simulink model "Reference_CVS"  (R2026a)
settings: Solver=ode1  StopTime=40
InitFcn:
  | %motor_control_init_m
  | %clear all
  | %close all
  | %clc
  | b=1e-8
  | StepSize = 1e-4;
  | N=1e-17;
  | 
  | VLV_0 =0;%120; %120
  | VA_0 = 0;%300; %300
  | VRV_0 = 0;%130;
  | VP_0 = 0;%500;
  | VLA_0 = 0;%20;
  | VV_0=5000;
  | VRA_0=0;
  | 
  | 
  | QLV_0 = 0;
  | QLA_0 = 0;
  | QP_0 = 0;
  | 
  | bh = 0;
  | th =0;
  | 
  | X_0 = [VLV_0 VA_0 VV_0 VP_0  VLA_0  VRA_0 VRV_0];
  | 
  | 
  | V0 = 10;
  | 
  | K1=.0004;%0.0001
  | K2=0.0009;%0.0009
  | KA=1;%1
  | C1=0.000000003;%0.0000003
  | lambda=6000;%3000
  | X_00 = [VLV_0 VA_0 VV_0 VRV_0];
  | 
  | r2 = 0.05/2;
  | A2 = pi*r2^2;
  | h2 = 0.63;
  | V2 = A2*h2;
  | 
  | 
  | r3 = 0.05/2;
  | A3 = pi*r3^2;
  | h3 = 0.63;
  | V3 = A3*h3;
  | 
  | 
  | rho = 997;
  | gg = 9.81;
  | %
  | init_min=0;
  | init_max=0;
  | %
  | PWM_Period =  StepSize;
  | PWM_Period_g1 = PWM_Period;
  | PWM_Period_g2 =PWM_Period;
  | PWM_Period_g3 = PWM_Period;
  | PWM_Period_g4 = PWM_Period;
  | PWM_Period_g5 = PWM_Period;
  | ... (+158 lines)
libraries: powerlib_meascontrol x12, simulink x8, cstblocks x6
(part 2 of 2)

== system Reference_CVS/Reference CVSs/eRV/eRVhf ==
  note: y = 0,0056x 2 - 0,6667x + 60
  Add18 : Sum
  Add19 : Sum
  Constant20 : Constant  Value=60
  Gain1 : Gain  Gain=1/100
  Gain2 : Gain  Gain=0.0056
  Gain3 : Gain  Gain=-0.6667
  PID : Subsystem  Commented=on
  Product15 : Product
  Scope : Scope
      settings: ActiveDisplayYMinimum=1.07059  ActiveDisplayYMaximum=1.42514
  Stair Generator : powerlib_meascontrol/Pulse & Signal Generators/Stair Generator  Commented=on  t=[0,50,100,150]  e=[3.25,3.5,3.75,4]  Ts=stepsize
      settings: SourceProductName=Simscape Electrical
  Stair Generator1 : powerlib_meascontrol/Pulse & Signal Generators/Stair Generator  Commented=on  t=[100,200,300,400]  e=[3.25,3.5,3.75,4]  Ts=stepsize
      settings: SourceProductName=Simscape Electrical
  Output : Outport
  wires:
  Stair Generator1/1 -> PID/1(s)
  Add19/1 -> Gain1/1
  Gain2/1 -> Add18/1
  Gain3/1 -> Add18/2
  [HR] -> Product15/1, Product15/2, Gain3/1
  Add18/1 -> Add19/1
  Product15/1 -> Gain2/1
  Constant20/1 -> Add19/2
  Gain1/1 -> Scope/1, Output/1

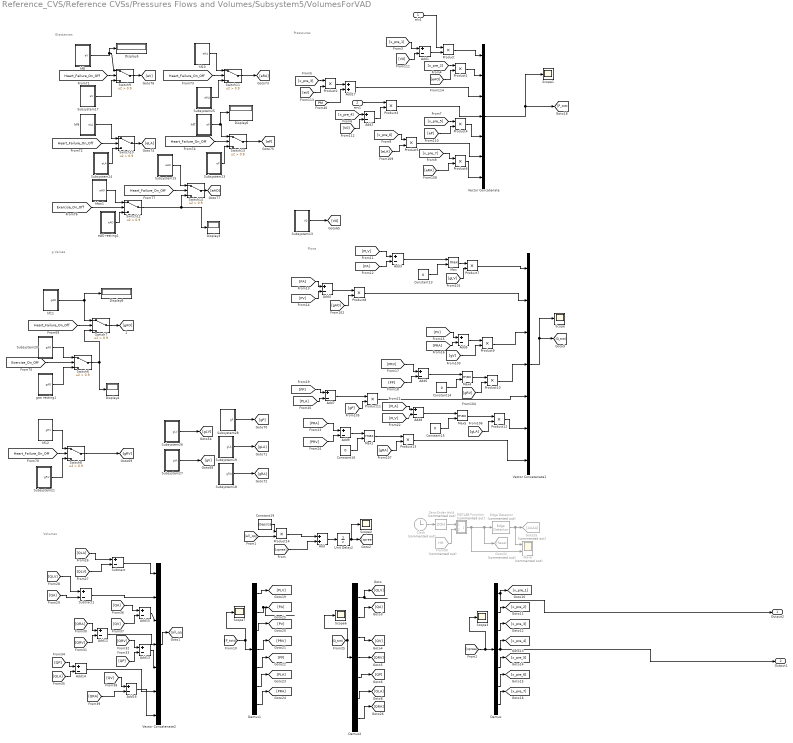
== system Reference_CVS/Reference CVSs/Pressures Flows and Volumes/Subsystem5/VolumesForVAD ==
  note: Elastances
  note: Presssures
  note: g Values
  note: Flows
  note: Volumes
  elv1 : Inport
  erv1 : Inport  Port=2
  Add : Sum
  Add{1..9,12..16} (14 alike) : Sum  Inputs=+-
  Add17 : Sum
  Clock : Clock  Commented=on
      settings: Decimation=10000000
  Constant{13..16} (4 alike) : Constant  Value=0
  Constant19 : Constant  Value=stepsize
  Demux : Demux  Outputs=7
  Demux1 : Demux  Outputs=7
  Demux2 : Demux  Outputs=7
  Display{3..6,8} (5 alike) : Display
  Edge Detector : powerlib_meascontrol/Logic/Edge Detector  Commented=on  model=Falling  ic=0  Ts=0
      settings: SourceProductName=Simscape Electrical
  From90 : From  Commented=on  GotoTag=HR  TagVisibility=global
  Goto32 : Goto  Commented=on  GotoTag=Reset
  Goto55 : Goto  Commented=on  GotoTag=AAAA
  MATLAB Function : MATLAB Function  Commented=on  TreatAsAtomicUnit=on
  Max{,1,4..5} (4 alike) : MinMax  Function=max  Inputs=2
  Product{,1..14} (15 alike) : Product
  Scope{,1..3,6..7} (6 alike) : Scope
      Scope settings: ActiveDisplayYMinimum=-554.9505  ActiveDisplayYMaximum=4972.61734
      Scope1 settings: ActiveDisplayYMinimum=60.37603  ActiveDisplayYMaximum=117.27305  DataLoggingVariableName=ScopeData2
      Scope2 settings: ActiveDisplayYMinimum=-34.04375  ActiveDisplayYMaximum=306.39376  DataLoggingVariableName=ScopeData4
      Scope3 settings: ActiveDisplayYMinimum=-652.22865  ActiveDisplayYMaximum=5628.02541  DataLoggingVariableName=ScopeData5
      Scope6 settings: ActiveDisplayYMinimum=-1063.20433  ActiveDisplayYMaximum=9460.42216  DataLoggingVariableName=ScopeData7
      Scope7 settings: ActiveDisplayYMinimum=-11.3052  ActiveDisplayYMaximum=174.2221  DataLoggingVariableName=ScopeData8
  Subsystem13 : Subsystem
  Subsystem15 : Subsystem
  Subsystem17 : Subsystem
  Subsystem18 : Subsystem
  Subsystem19 : Subsystem
  Subsystem20 : Subsystem
  Subsystem21 : Subsystem
  Subsystem23 : Subsystem
  Subsystem24 : Subsystem
  Subsystem25 : Subsystem
  Subsystem26 : Subsystem
  Subsystem27 : Subsystem
  Subsystem28 : Subsystem
  Subtract : Sum  Inputs=+-
  Subtract1 : Sum  Inputs=+-
  Switch{6..14} (9 alike) : Switch  Criteria=u2 > Threshold  Threshold=0.9  SaturateOnIntegerOverflow=off  InputSameDT=off
  Unit Delay2 : UnitDelay  InitialCondition=X_0  SampleTime=-1
  Vector Concatenate : Concatenate  NumInputs=7
  Vector Concatenate1 : Concatenate  NumInputs=7
  Vector Concatenate2 : Concatenate  NumInputs=7
  Wave : Scope  Commented=on  NumInputPorts=2
      settings: ActiveDisplayYMinimum=-0.125  ActiveDisplayYMaximum=1.125  DataLoggingVariableName=ScopeData10
  Zero-Order Hold : ZeroOrderHold  Commented=on  SampleTime=-1
  eAO resting1 : Subsystem
  gao resting1 : Subsystem
  hf10 : Subsystem
  hf11 : Subsystem
  hf12 : Subsystem
  hf7 : Subsystem
  hf8 : Subsystem
  hf9 : Subsystem
  hfao1 : Subsystem
  Output2 : Outport
  Output1 : Outport  Port=2
  wires:
  Add/1 -> Unit Delay2/1
  Demux1/2 -> [PA]
  Product4/1 -> Vector Concatenate/5
  [QA] -> Add15/1
  Add1/1 -> Product/2
  [P_tott] -> Demux1/1, Scope7/1
  [QRV] -> Add13/1
  Demux/3 -> [x_pre_3]
  [x_pre_7] -> Product6/1
  Product13/1 -> Vector Concatenate1/7
  Demux1/6 -> [PLA]
  [PP] -> Add6/2
  Demux2/2 -> [QA]
  Demux1/4 -> [PRV]
  Product14/1 -> Add/1
  Add9/1 -> Max1/1
  elv1/1 -> Product/1
  Demux2/6 -> [QLA]
  Product/1 -> Vector Concatenate/1
  Constant13/1 -> Max/2
  [QV] -> Add16/1
  [PLV] -> Add8/2
  Constant15/1 -> Max5/2
  [PLV] -> Add3/1
  Max5/1 -> Product12/1
  Demux1/7 -> [PRA]
  [PRV] -> Add6/1
  [PA] -> Add4/1
  Demux1/1 -> [PLV]
  [QRA] -> Add12/1
  [Heart_Failure_On_Off] -> Switch7/2
  [QV] -> Add15/2
  Product10/1 -> Vector Concatenate1/4
  Add5/1 -> Product9/1
  Subsystem21/1(gRV) -> Switch8/3
  Product11/1 -> Vector Concatenate1/5
  [PLA] -> Add8/1
  Add6/1 -> Max4/1
  [PV] -> Add5/1
  [x_pre_4] -> Add2/1
  [QA] -> Subtract1/2
  [x_pre_6] -> Product5/1
  erv1/1 -> Product3/1
  Demux2/1 -> [QLV]
  [x_pre_1] -> Add1/1
  [QRA] -> Add16/2
  [QLA] -> Subtract/1
  Max1/1 -> Product13/1
  Subsystem19/1(gLA) -> [gLA]
  [QLV] -> Subtract1/1
  [Heart_Failure_On_Off] -> Switch10/2
  Add13/1 -> Vector Concatenate2/5
  Add17/1 -> Vector Concatenate/3
  [Heart_Failure_On_Off] -> Switch14/2
  Product9/1 -> Vector Concatenate1/3
  Product2/1 -> Add17/1
  Vector Concatenate/1 -> Scope1/1, [P_tott]
  Unit Delay2/1 -> [xpree], Scope2/1
  Add12/1 -> Vector Concatenate2/4
  hf12/1(gRV) -> Switch8/1
  [x_pre_3] -> Product2/1
  [QLV] -> Subtract/2
  Product3/1 -> Vector Concatenate/4
  [eP] -> Product4/2
  [V0] -> Add2/2
  [gAO] -> Product8/2
  Vector Concatenate1/1 -> Scope/1, [Q_tott]
  Product12/1 -> Vector Concatenate1/6
  [gLA] -> Product12/2
  [gRA] -> Product13/2
  [eV] -> Product2/2
  [eRA] -> Product6/2
  [xpree] -> Add/2
  [gP] -> Product11/2
  Max/1 -> Product7/1
  MATLAB Function/1(y) -> Goto32/1, Edge Detector/1, Wave/2
  Product5/1 -> Vector Concatenate/6
  From90/1 -> MATLAB Function/2(HR)
  [x_pre_5] -> Product4/1
  Switch9/1 -> [eV]
  [gRV] -> Product10/2
  Product8/1 -> Vector Concatenate1/2
  Demux/7 -> [x_pre_7]
  Add8/1 -> Max5/1
  Demux2/7 -> [QRA]
  Vector Concatenate2/1 -> [all_qq]
  Zero-Order Hold/1 -> MATLAB Function/1(u)
  Add15/1 -> Vector Concatenate2/3
  Demux2/5 -> [QP]
  Demux2/4 -> [QRV]
  hfao1/1(eAO) -> Switch12/1
  Add16/1 -> Vector Concatenate2/7
  Max4/1 -> Product10/1
  Edge Detector/1 -> Goto55/1, Wave/1
  Demux/6 -> [x_pre_6]
  Demux/1 -> Output2/1, [x_pre_1]
  [PRA] -> Add9/1
  hf8/1(eV) -> Switch9/1, Display5/1
  Subsystem13/1(V0) -> [V0]
  Subsystem15/1(eAO) -> Switch14/1
  Subsystem27/1(gVt) -> [gV]
  Demux/2 -> [x_pre_2]
  Subsystem26/1(gLV) -> [gLV]
  Add4/1 -> Product8/1
  Add14/1 -> Vector Concatenate2/6
  Demux1/5 -> [PP]
  [PRV] -> Add9/2
  Subtract1/1 -> Vector Concatenate2/2
  [PRA] -> Add5/2
  [QP] -> Add13/2
  [PV] -> Add4/2
  [gV] -> Product9/2
  Switch13/1 -> [eP]
  Clock/1 -> Zero-Order Hold/1
  Switch10/1 -> [eLA]
  [Heart_Failure_On_Off] -> Switch9/2
  [x_pre_2] -> Product1/1
  Add3/1 -> Max/1
  Demux/4 -> Output1/1, [x_pre_4]
  [Heart_Failure_On_Off] -> Switch13/2
  Switch11/1 -> [eRA]
  Switch12/1 -> Switch14/3, Display3/1
  Product7/1 -> Vector Concatenate1/1
  gao resting1/1(gAO) -> Switch6/3
  Switch6/1 -> Display4/1, Switch7/3
  Demux/5 -> [x_pre_5]
  [QP] -> Add14/1
  Constant19/1 -> Product14/1
  Subsystem24/1(eLA) -> Switch10/3
  [PA] -> Add3/2
  ? -> ?
  [PLA] -> Add7/2
  [Heart_Failure_On_Off] -> Switch8/2
  hf11/1(gAO) -> Switch7/1, Display8/1
  Subsystem23/1(eP) -> Switch13/3
  Subsystem17/1(eV) -> Switch9/3
  [eLA] -> Product5/2
  Subsystem20/1(gAO) -> Switch6/1
  Add7/1 -> Product11/1
  [all_qq] -> Product14/2
  Switch14/1 -> [eAO]
  Switch8/1 -> [gRV]
  Subsystem18/1(gRA) -> [gRA]
  Switch7/1 -> [gAO]
  [xpree] -> Demux/1, Scope3/1
  Subsystem28/1(gP) -> [gP]
  Product1/1 -> Vector Concatenate/2
  [PM] -> Add17/2
  hf10/1(eRA) -> Switch11/1
  [QLA] -> Add14/2
  [Exercise_On_Off] -> Switch12/2
  Subtract/1 -> Vector Concatenate2/1
  Demux2/3 -> [QV]
  eAO resting1/1(eAO) -> Switch12/3
  Product6/1 -> Vector Concatenate/7
  [V0] -> Add1/2
  [Heart_Failure_On_Off] -> Switch11/2
  Subsystem25/1(eRA) -> Switch11/3
  [PP] -> Add7/1
  [eAO] -> Product1/2
  Constant14/1 -> Max4/2
  Add2/1 -> Product3/2
  [Q_tott] -> Scope6/1, Demux2/1
  [Exercise_On_Off] -> Switch6/2
  hf9/1(eLA) -> Switch10/1
  Constant16/1 -> Max1/2
  [gLV] -> Product7/2
  [QRV] -> Add12/2
  hf7/1(eP) -> Switch13/1, Display6/1
  Demux1/3 -> [PV]

== system Reference_CVS/Reference CVSs/eLV/LV_e_min/Real_CLV ==
  note: y = 0,2444x 2 - 30,667x + 2560
      | R² = 1
  Add18 : Sum
  Add19 : Sum
  Constant20 : Constant  Value=25600
  Gain : Gain  Gain=1/100
  Gain2 : Gain  Gain=2.444
  Gain3 : Gain  Gain=- 306.67
  Product15 : Product
  C_LV : Outport
  wires:
  Gain/1 -> C_LV/1
  Add18/1 -> Add19/1
  Gain3/1 -> Add18/2
  Product15/1 -> Gain2/1
  Constant20/1 -> Add19/2
  Gain2/1 -> Add18/1
  [HR] -> Product15/1, Product15/2, Gain3/1
  Add19/1 -> Gain/1

== system Reference_CVS/Reference CVSs/eLV/LV_e_min/Subsystem1 ==
  note: y = 0,0446x 2 - 6,3542x + 365,75
      | R² = 1
  Add18 : Sum
  Add19 : Sum
  Constant20 : Constant  Value=365.75
  Gain2 : Gain  Gain=0.0446
  Gain3 : Gain  Gain=- 6.3542
  Product15 : Product
  C_LV : Outport
  wires:
  Add19/1 -> C_LV/1
  [HR] -> Gain3/1, Product15/2, Product15/1
  Gain2/1 -> Add18/1
  Constant20/1 -> Add19/2
  Product15/1 -> Gain2/1
  Gain3/1 -> Add18/2
  Add18/1 -> Add19/1

== system Reference_CVS/Reference CVSs/eLV/LV_e_min/Subsystem2 ==
  note: y = -0,0175x 2 + 5,625x - 264,5
      | R² = 1
  note: y = 0,0011x 2 - 0,4292x + 39,85
      | R² = 1
  note: y = 0,0108x 2 - 4,2917x + 398,5
      | R² = 1
  Add18 : Sum
  Add19 : Sum
  Constant20 : Constant  Value=398.5
  Gain : Gain  Gain=1/10000
  Gain2 : Gain  Gain=0.0108
  Gain3 : Gain  Gain=-4.2917
  Product15 : Product
  Scope : Scope
      settings: ActiveDisplayYMinimum=-0.00112  ActiveDisplayYMaximum=0.02012  DataLoggingVariableName=ScopeData2
  B_LV : Outport
  wires:
  Gain/1 -> B_LV/1, Scope/1
  Add19/1 -> Gain/1
  [HR] -> Gain3/1, Product15/2, Product15/1
  Gain2/1 -> Add18/1
  Constant20/1 -> Add19/2
  Product15/1 -> Gain2/1
  Gain3/1 -> Add18/2
  Add18/1 -> Add19/1

== system Reference_CVS/Reference CVSs/eLV/LV_e_min/Subsystem5 ==
  note: y = -0,0033x 2 + 0,4333x - 2
      | R² = 1
  Add18 : Sum
  Add19 : Sum
  Constant20 : Constant  Value=-20
  Gain : Gain  Gain=1/10000
  Gain2 : Gain  Gain=-0.0333
  Gain3 : Gain  Gain=4.333
  Product15 : Product
  Scope : Scope
      settings: ActiveDisplayYMinimum=-0.00112  ActiveDisplayYMaximum=0.02012  DataLoggingVariableName=ScopeData2
  B_LV_HF : Outport
  wires:
  Add18/1 -> Add19/1
  Gain3/1 -> Add18/2
  Product15/1 -> Gain2/1
  Constant20/1 -> Add19/2
  Gain2/1 -> Add18/1
  [HR] -> Product15/1, Product15/2, Gain3/1
  Add19/1 -> Gain/1
  Gain/1 -> Scope/1, B_LV_HF/1

== system Reference_CVS/Reference CVSs/eLV/LV_e_min/resting ==
  note: y = -4,3333x + 440
  Add19 : Sum
  Constant20 : Constant  Value=440
  Gain : Gain  Gain=1/10000
  Gain3 : Gain  Gain=-4.3333
  Scope : Scope
      settings: ActiveDisplayYMinimum=-0.00112  ActiveDisplayYMaximum=0.02012  DataLoggingVariableName=ScopeData2
  B_LV : Outport
  wires:
  Gain3/1 -> Add19/1
  Constant20/1 -> Add19/2
  [insan] -> Gain3/1
  Add19/1 -> Gain/1
  Gain/1 -> Scope/1, B_LV/1

== system Reference_CVS/Reference CVSs/eLV/eLV1/PID ==
  s : Inport
  LTI System : cstblocks/LTI System  sys=tfa  IC=[]
  PID Controller : simulink/Continuous/PID Controller  Controller=PID  Form=Parallel  TimeDomain=Continuous-time  SampleTime=-1  IntegratorMethod=Forward Euler  FilterMethod=Forward Euler  ControllerParametersSource=internal  P=0  I=0.336541519886425  D=0  UseFilter=on  N=100  TunerSelectOption=Transfer Function Based (PID Tuner App)  InitialConditionSource=internal  InitialConditionForIntegrator=0  InitialConditionForFilter=0  DifferentiatorICPrevScaledInput=0  ExternalReset=none  TrackingMode=off  Kt=1  LimitOutput=off  UpperSaturationLimit=inf  LowerSaturationLimit=-inf  LinearizeAsGain=on  AntiWindupMode=none  Kb=1  POutMin=[]  POutMax=[]  IOutMin=[]  IOutMax=[]  DOutMin=[]  DOutMax=[]  NOutMin=[]  NOutMax=[]  SumOutMin=[]  SumOutMax=[]  SaturationOutMin=[]  SaturationOutMax=[]  PParamMin=[]  PParamMax=[]  IParamMin=[]  IParamMax=[]  DParamMin=[]  DParamMax=[]  NParamMin=[]  NParamMax=[]  KbParamMin=[]  KbParamMax=[]  KtParamMin=[]  KtParamMax=[]  KbOutMin=[]  KbOutMax=[]  KtOutMin=[]  KtOutMax=[]  IntegratorOutMin=[]  IntegratorOutMax=[]  FilterOutMin=[]  FilterOutMax=[]  SumI1OutMin=[]  SumI1OutMax=[]  SumI2OutMin=[]  SumI2OutMax=[]  SumI3OutMin=[]  SumI3OutMax=[]  SumI4OutMin=[]  SumI4OutMax=[]  SumDOutMin=[]  SumDOutMax=[]  DifferentiatorOutMin=[]  DifferentiatorOutMax=[]  FilterDiffOutCoefMin=[]  FilterDiffOutCoefMax=[]  ReciprocalOutMin=[]  ReciprocalOutMax=[]  SumDenOutMin=[]  SumDenOutMax=[]  SumNumOutMin=[]  SumNumOutMax=[]  DivideOutMin=[]  DivideOutMax=[]  IntegratorContinuousStateAttributes=''  IntegratorStateMustResolveToSignalObject=off  IntegratorRTWStateStorageClass=Auto  FilterContinuousStateAttributes=''  FilterStateMustResolveToSignalObject=off  FilterRTWStateStorageClass=Auto  ParallelPVariant=InternalParameters  IdealPVariant=Disabled  IVariant=InternalParameters  DVariant=InternalParameters  IntegratorVariant=Continuous  SatVariant=Disabled  AWVariant=Passthrough  PCopyVariant=Disabled  TRVariant=Disabled  FdbkBlocksVariant=Forward  IdealPFdbkVariant=Disabled  SatFdbkVariant=Disabled  DerivativeFilterVariant=ContFilter  NVariant=InternalParameters  NCopyVariant=Disabled  FilterICVariant=InternalICsFilter  IntegratorICVariant=InternalICs  ExternalResetVariant=Disabled  TRSumVariant=Passthrough  SumFdbkVariant=Disabled  SumVariant=Sum_PID
  Sum1 : Sum  Inputs=|+-
  To Workspace : ToWorkspace  VariableName=input  SampleTime=-1
  To Workspace1 : ToWorkspace  VariableName=output  SampleTime=-1
  E : Outport  VectorParamsAs1DForOutWhenUnconnected=off
  wires:
  PID Controller/1 -> To Workspace/1, LTI System/1
  s/1 -> Sum1/1
  Sum1/1 -> PID Controller/1
  LTI System/1 -> Sum1/2, E/1, To Workspace1/1

== system Reference_CVS/Reference CVSs/eRV/RV_e_min/c_RV ==
  note: y = 0,0167x 2 - 3,3333x + 290
  Add18 : Sum
  Add19 : Sum
  Constant20 : Constant  Value=290
  Gain2 : Gain  Gain=0.0167
  Gain3 : Gain  Gain=-3.3333
  PID : Subsystem  Commented=on
  Product15 : Product
  Scope : Scope
      settings: ActiveDisplayYMinimum=1.07059  ActiveDisplayYMaximum=1.42514
  Stair Generator : powerlib_meascontrol/Pulse & Signal Generators/Stair Generator  Commented=on  t=[0,50,100,150]  e=[3.25,3.5,3.75,4]  Ts=stepsize
      settings: SourceProductName=Simscape Electrical
  Stair Generator1 : powerlib_meascontrol/Pulse & Signal Generators/Stair Generator  Commented=on  t=[100,200,300,400]  e=[3.25,3.5,3.75,4]  Ts=stepsize
      settings: SourceProductName=Simscape Electrical
  Output : Outport
  wires:
  Add19/1 -> Output/1, Scope/1
  Constant20/1 -> Add19/2
  Product15/1 -> Gain2/1
  Add18/1 -> Add19/1
  [HR] -> Gain3/1, Product15/2, Product15/1
  Gain3/1 -> Add18/2
  Gain2/1 -> Add18/1
  Stair Generator1/1 -> PID/1(s)

== system Reference_CVS/Reference CVSs/eRV/RV_e_min/real_c_RV ==
  note: y = - 333,33x + 110000
      | R² = 1
  Add19 : Sum
  Constant20 : Constant  Value=110000
  Gain1 : Gain  Gain=1/1000
  Gain3 : Gain  Gain=-333.33
  PID : Subsystem  Commented=on
  Scope : Scope
      settings: ActiveDisplayYMinimum=1.07059  ActiveDisplayYMaximum=1.42514
  Stair Generator : powerlib_meascontrol/Pulse & Signal Generators/Stair Generator  Commented=on  t=[0,50,100,150]  e=[3.25,3.5,3.75,4]  Ts=stepsize
      settings: SourceProductName=Simscape Electrical
  Stair Generator1 : powerlib_meascontrol/Pulse & Signal Generators/Stair Generator  Commented=on  t=[100,200,300,400]  e=[3.25,3.5,3.75,4]  Ts=stepsize
      settings: SourceProductName=Simscape Electrical
  Output : Outport
  wires:
  Gain1/1 -> Scope/1, Output/1
  Stair Generator1/1 -> PID/1(s)
  [HR] -> Gain3/1
  Gain3/1 -> Add19/1
  Constant20/1 -> Add19/2
  Add19/1 -> Gain1/1

== system Reference_CVS/Reference CVSs/eRV/Subsystem2/k_0 ==
  note: y = -0,0042x 2 - 0,0417x + 257,5
      | R² = 1
  In1 : Inport
  Add4 : Sum
  Add5 : Sum
  Constant4 : Constant  Value=257.5
  Gain : Gain  Gain=-0.0041
  Gain1 : Gain  Gain=-0.0417
  Multiply : Gain  Gain=1/1000
  Product8 : Product
  Out1 : Outport
  wires:
  Multiply/1 -> Out1/1
  Add5/1 -> Multiply/1
  Constant4/1 -> Add5/2
  Gain/1 -> Add4/1
  Gain1/1 -> Add4/2
  Product8/1 -> Gain/1
  In1/1 -> Product8/1, Product8/2, Gain1/1
  Add4/1 -> Add5/1

== system Reference_CVS/Reference CVSs/eRV/Subsystem2/k_1 ==
  note: y = 0,0158x 2 - 5,0417x + 445,5
      | R² = 1
  In1 : Inport
  Add6 : Sum
  Add7 : Sum
  Constant7 : Constant  Value=445.5
  Gain2 : Gain  Gain=0.0158
  Gain3 : Gain  Gain=-5.0417
  Multiply : Gain  Gain=1/1000
  Product10 : Product
  Out1 : Outport
  wires:
  Multiply/1 -> Out1/1
  Add7/1 -> Multiply/1
  Product10/1 -> Gain2/1
  Add6/1 -> Add7/1
  Gain3/1 -> Add6/2
  In1/1 -> Product10/1, Product10/2, Gain3/1
  Gain2/1 -> Add6/1
  Constant7/1 -> Add7/2

== system Reference_CVS/Reference CVSs/eRV/eRV2/PID ==
  s : Inport
  LTI System : cstblocks/LTI System  sys=tfa  IC=[]
  PID Controller : simulink/Continuous/PID Controller  Controller=PID  Form=Parallel  TimeDomain=Continuous-time  SampleTime=-1  IntegratorMethod=Forward Euler  FilterMethod=Forward Euler  ControllerParametersSource=internal  P=0  I=0.336541519886425  D=0  UseFilter=on  N=100  TunerSelectOption=Transfer Function Based (PID Tuner App)  InitialConditionSource=internal  InitialConditionForIntegrator=0  InitialConditionForFilter=0  DifferentiatorICPrevScaledInput=0  ExternalReset=none  TrackingMode=off  Kt=1  LimitOutput=off  UpperSaturationLimit=inf  LowerSaturationLimit=-inf  LinearizeAsGain=on  AntiWindupMode=none  Kb=1  POutMin=[]  POutMax=[]  IOutMin=[]  IOutMax=[]  DOutMin=[]  DOutMax=[]  NOutMin=[]  NOutMax=[]  SumOutMin=[]  SumOutMax=[]  SaturationOutMin=[]  SaturationOutMax=[]  PParamMin=[]  PParamMax=[]  IParamMin=[]  IParamMax=[]  DParamMin=[]  DParamMax=[]  NParamMin=[]  NParamMax=[]  KbParamMin=[]  KbParamMax=[]  KtParamMin=[]  KtParamMax=[]  KbOutMin=[]  KbOutMax=[]  KtOutMin=[]  KtOutMax=[]  IntegratorOutMin=[]  IntegratorOutMax=[]  FilterOutMin=[]  FilterOutMax=[]  SumI1OutMin=[]  SumI1OutMax=[]  SumI2OutMin=[]  SumI2OutMax=[]  SumI3OutMin=[]  SumI3OutMax=[]  SumI4OutMin=[]  SumI4OutMax=[]  SumDOutMin=[]  SumDOutMax=[]  DifferentiatorOutMin=[]  DifferentiatorOutMax=[]  FilterDiffOutCoefMin=[]  FilterDiffOutCoefMax=[]  ReciprocalOutMin=[]  ReciprocalOutMax=[]  SumDenOutMin=[]  SumDenOutMax=[]  SumNumOutMin=[]  SumNumOutMax=[]  DivideOutMin=[]  DivideOutMax=[]  IntegratorContinuousStateAttributes=''  IntegratorStateMustResolveToSignalObject=off  IntegratorRTWStateStorageClass=Auto  FilterContinuousStateAttributes=''  FilterStateMustResolveToSignalObject=off  FilterRTWStateStorageClass=Auto  ParallelPVariant=InternalParameters  IdealPVariant=Disabled  IVariant=InternalParameters  DVariant=InternalParameters  IntegratorVariant=Continuous  SatVariant=Disabled  AWVariant=Passthrough  PCopyVariant=Disabled  TRVariant=Disabled  FdbkBlocksVariant=Forward  IdealPFdbkVariant=Disabled  SatFdbkVariant=Disabled  DerivativeFilterVariant=ContFilter  NVariant=InternalParameters  NCopyVariant=Disabled  FilterICVariant=InternalICsFilter  IntegratorICVariant=InternalICs  ExternalResetVariant=Disabled  TRSumVariant=Passthrough  SumFdbkVariant=Disabled  SumVariant=Sum_PID
  Sum1 : Sum  Inputs=|+-
  To Workspace : ToWorkspace  VariableName=input  SampleTime=-1
  To Workspace1 : ToWorkspace  VariableName=output  SampleTime=-1
  E : Outport  VectorParamsAs1DForOutWhenUnconnected=off
  wires:
  LTI System/1 -> To Workspace1/1, E/1, Sum1/2
  Sum1/1 -> PID Controller/1
  s/1 -> Sum1/1
  PID Controller/1 -> LTI System/1, To Workspace/1

== system Reference_CVS/Reference CVSs/eRV/eRVhf/PID ==
  s : Inport
  LTI System : cstblocks/LTI System  sys=tfa  IC=[]
  PID Controller : simulink/Continuous/PID Controller  Controller=PID  Form=Parallel  TimeDomain=Continuous-time  SampleTime=-1  IntegratorMethod=Forward Euler  FilterMethod=Forward Euler  ControllerParametersSource=internal  P=0  I=0.336541519886425  D=0  UseFilter=on  N=100  TunerSelectOption=Transfer Function Based (PID Tuner App)  InitialConditionSource=internal  InitialConditionForIntegrator=0  InitialConditionForFilter=0  DifferentiatorICPrevScaledInput=0  ExternalReset=none  TrackingMode=off  Kt=1  LimitOutput=off  UpperSaturationLimit=inf  LowerSaturationLimit=-inf  LinearizeAsGain=on  AntiWindupMode=none  Kb=1  POutMin=[]  POutMax=[]  IOutMin=[]  IOutMax=[]  DOutMin=[]  DOutMax=[]  NOutMin=[]  NOutMax=[]  SumOutMin=[]  SumOutMax=[]  SaturationOutMin=[]  SaturationOutMax=[]  PParamMin=[]  PParamMax=[]  IParamMin=[]  IParamMax=[]  DParamMin=[]  DParamMax=[]  NParamMin=[]  NParamMax=[]  KbParamMin=[]  KbParamMax=[]  KtParamMin=[]  KtParamMax=[]  KbOutMin=[]  KbOutMax=[]  KtOutMin=[]  KtOutMax=[]  IntegratorOutMin=[]  IntegratorOutMax=[]  FilterOutMin=[]  FilterOutMax=[]  SumI1OutMin=[]  SumI1OutMax=[]  SumI2OutMin=[]  SumI2OutMax=[]  SumI3OutMin=[]  SumI3OutMax=[]  SumI4OutMin=[]  SumI4OutMax=[]  SumDOutMin=[]  SumDOutMax=[]  DifferentiatorOutMin=[]  DifferentiatorOutMax=[]  FilterDiffOutCoefMin=[]  FilterDiffOutCoefMax=[]  ReciprocalOutMin=[]  ReciprocalOutMax=[]  SumDenOutMin=[]  SumDenOutMax=[]  SumNumOutMin=[]  SumNumOutMax=[]  DivideOutMin=[]  DivideOutMax=[]  IntegratorContinuousStateAttributes=''  IntegratorStateMustResolveToSignalObject=off  IntegratorRTWStateStorageClass=Auto  FilterContinuousStateAttributes=''  FilterStateMustResolveToSignalObject=off  FilterRTWStateStorageClass=Auto  ParallelPVariant=InternalParameters  IdealPVariant=Disabled  IVariant=InternalParameters  DVariant=InternalParameters  IntegratorVariant=Continuous  SatVariant=Disabled  AWVariant=Passthrough  PCopyVariant=Disabled  TRVariant=Disabled  FdbkBlocksVariant=Forward  IdealPFdbkVariant=Disabled  SatFdbkVariant=Disabled  DerivativeFilterVariant=ContFilter  NVariant=InternalParameters  NCopyVariant=Disabled  FilterICVariant=InternalICsFilter  IntegratorICVariant=InternalICs  ExternalResetVariant=Disabled  TRSumVariant=Passthrough  SumFdbkVariant=Disabled  SumVariant=Sum_PID
  Sum1 : Sum  Inputs=|+-
  To Workspace : ToWorkspace  VariableName=input  SampleTime=-1
  To Workspace1 : ToWorkspace  VariableName=output  SampleTime=-1
  E : Outport  VectorParamsAs1DForOutWhenUnconnected=off
  wires:
  LTI System/1 -> To Workspace1/1, E/1, Sum1/2
  Sum1/1 -> PID Controller/1
  s/1 -> Sum1/1
  PID Controller/1 -> LTI System/1, To Workspace/1

== system Reference_CVS/Reference CVSs/Pressures Flows and Volumes/Subsystem5/VolumesForVAD/Subsystem13 ==
  note: y = 0,1944x 2 - 28,333x + 1100
  Add{1..2,18..19} (4 alike) : Sum
  Constant1 : Constant  Value=2750
  Constant20 : Constant  Value=1100
  Display : Display
  Gain : Gain  Gain=1/10
  Gain1 : Gain  Gain=1/1000
  Gain2 : Gain  Gain=0.1944
  Gain3 : Gain  Gain=-28.333
  Gain4 : Gain  Gain=-0.4167
  Gain5 : Gain  Gain=145.83
  Product1 : Product
  Product15 : Product
  Scope : Scope
      settings: ActiveDisplayYMinimum=8.99968  ActiveDisplayYMaximum=10.99968  DataLoggingVariableName=ScopeData2
  Scope1 : Scope
      settings: ActiveDisplayYMinimum=8.99968  ActiveDisplayYMaximum=10.99968
  Switch : Switch  Criteria=u2 > Threshold  SaturateOnIntegerOverflow=off  InputSameDT=off
  V0 : Outport
  wires:
  Switch/1 -> V0/1, Display/1
  [Heart_Failure_On_Off] -> Switch/2
  Add2/1 -> Gain1/1
  Add1/1 -> Add2/1
  Gain5/1 -> Add1/2
  Product1/1 -> Gain4/1
  Constant1/1 -> Add2/2
  Gain4/1 -> Add1/1
  [HR] -> Product1/1, Product1/2, Gain5/1
  Gain1/1 -> Scope1/1, Switch/3
  Gain/1 -> Scope/1, Switch/1
  [HR] -> Gain3/1, Product15/2, Product15/1
  Gain2/1 -> Add18/1
  Constant20/1 -> Add19/2
  Product15/1 -> Gain2/1
  Gain3/1 -> Add18/2
  Add18/1 -> Add19/1
  Add19/1 -> Gain/1

== system Reference_CVS/Reference CVSs/Pressures Flows and Volumes/Subsystem5/VolumesForVAD/Subsystem15 ==
  note: y = -0,0278x 2 + 5,8333x - 150
  Add18 : Sum
  Add19 : Sum
  Constant20 : Constant  Value=-150
  Gain2 : Gain  Gain=-0.0278
  Gain3 : Gain  Gain=5.8333
  Multiply : Gain  Gain=1/100
  Product15 : Product
  Scope : Scope
      settings: ActiveDisplayYMinimum=0.50527  ActiveDisplayYMaximum=0.53249  DataLoggingVariableName=ScopeData2
  eAO : Outport
  wires:
  Multiply/1 -> Scope/1, eAO/1
  [HR] -> Gain3/1, Product15/2, Product15/1
  Gain2/1 -> Add18/1
  Constant20/1 -> Add19/2
  Product15/1 -> Gain2/1
  Gain3/1 -> Add18/2
  Add18/1 -> Add19/1
  Add19/1 -> Multiply/1

== system Reference_CVS/Reference CVSs/Pressures Flows and Volumes/Subsystem5/VolumesForVAD/Subsystem17 ==
  note: y = -0,0033x 2 + 0,8667x - 16
  Add18 : Sum
  Add19 : Sum
  Constant20 : Constant  Value=-16
  Gain1 : Gain  Gain=1/10000
  Gain2 : Gain  Gain=-0.0033
  Gain3 : Gain  Gain=0.8667
  Product15 : Product
  Scope : Scope
      settings: ActiveDisplayYMinimum=0.00132  ActiveDisplayYMaximum=0.00154  DataLoggingVariableName=ScopeData2
  eV : Outport
  wires:
  Add18/1 -> Add19/1
  Gain3/1 -> Add18/2
  Product15/1 -> Gain2/1
  Constant20/1 -> Add19/2
  Gain2/1 -> Add18/1
  [HR] -> Product15/1, Product15/2, Gain3/1
  Add19/1 -> Gain1/1
  Gain1/1 -> Scope/1, eV/1

== system Reference_CVS/Reference CVSs/Pressures Flows and Volumes/Subsystem5/VolumesForVAD/Subsystem18 ==
  note: y = 0,0167x 2 - 5,8333x + 1290
      | R² = 1
  Add19 : Sum
  Constant20 : Constant  Value=1150
  Gain3 : Gain  Gain=-2.5
  Scope : Scope
      settings: ActiveDisplayYMinimum=900  ActiveDisplayYMaximum=1100  DataLoggingVariableName=ScopeData2
  gRA : Outport
  wires:
  Gain3/1 -> Add19/1
  Add19/1 -> gRA/1, Scope/1
  [HR] -> Gain3/1
  Constant20/1 -> Add19/2

== system Reference_CVS/Reference CVSs/Pressures Flows and Volumes/Subsystem5/VolumesForVAD/Subsystem19 ==
  note: y = 0,0167x 2 - 5,8333x + 1290
      | R² = 1
  note: y = - 5x + 1300R² = 1
  Add19 : Sum
  Constant20 : Constant  Value=1300
  Gain3 : Gain  Gain=-5
  Scope : Scope
      settings: ActiveDisplayYMinimum=900  ActiveDisplayYMaximum=1100  DataLoggingVariableName=ScopeData2
  gLA : Outport
  wires:
  Gain3/1 -> Add19/1
  Constant20/1 -> Add19/2
  [HR] -> Gain3/1
  Add19/1 -> Scope/1, gLA/1

== system Reference_CVS/Reference CVSs/Pressures Flows and Volumes/Subsystem5/VolumesForVAD/Subsystem20 ==
  note: y = 0,0058x 2 + 1,4583x - 18,5
  Add18 : Sum
  Add19 : Sum
  Constant20 : Constant  Value=-18.5
  Gain1 : Gain  Gain=1/100
  Gain2 : Gain  Gain=0.0058
  Gain3 : Gain  Gain=1.4583
  Product15 : Product
  Scope : Scope
      settings: ActiveDisplayYMinimum=0.88246  ActiveDisplayYMaximum=1.08246  DataLoggingVariableName=ScopeData2
  gAO : Outport
  wires:
  Add18/1 -> Add19/1
  Gain3/1 -> Add18/2
  Product15/1 -> Gain2/1
  Constant20/1 -> Add19/2
  Gain2/1 -> Add18/1
  [HR] -> Product15/1, Product15/2, Gain3/1
  Add19/1 -> Gain1/1
  Gain1/1 -> Scope/1, gAO/1

== system Reference_CVS/Reference CVSs/Pressures Flows and Volumes/Subsystem5/VolumesForVAD/Subsystem21 ==
  note: y = 0,0742x 2 - 10,958x + 600,5
  Add18 : Sum
  Add19 : Sum
  Constant20 : Constant  Value=600.5
  Gain : Gain
  Gain2 : Gain  Gain=0.0742
  Gain3 : Gain  Gain=-10.958
  Product15 : Product
  Scope : Scope
      settings: ActiveDisplayYMinimum=109.99968  ActiveDisplayYMaximum=309.99968  DataLoggingVariableName=ScopeData2
  gRV : Outport
  wires:
  Add19/1 -> Gain/1
  [HR] -> Gain3/1, Product15/2, Product15/1
  Gain2/1 -> Add18/1
  Constant20/1 -> Add19/2
  Product15/1 -> Gain2/1
  Gain3/1 -> Add18/2
  Add18/1 -> Add19/1
  Gain/1 -> gRV/1, Scope/1

== system Reference_CVS/Reference CVSs/Pressures Flows and Volumes/Subsystem5/VolumesForVAD/Subsystem23 ==
  note: y = 0,1417x 2 - 24,583x + 2165
  Add18 : Sum
  Add19 : Sum
  Constant20 : Constant  Value=2165
  Gain : Gain  Gain=1/10000
  Gain2 : Gain  Gain=0.1417
  Gain3 : Gain  Gain=-24.583
  Product15 : Product
  Scope : Scope
      settings: ActiveDisplayYMinimum=0.01994  ActiveDisplayYMaximum=0.21994  DataLoggingVariableName=ScopeData2
  eP : Outport
  wires:
  Add19/1 -> Gain/1
  [HR] -> Gain3/1, Product15/2, Product15/1
  Gain2/1 -> Add18/1
  Constant20/1 -> Add19/2
  Product15/1 -> Gain2/1
  Gain3/1 -> Add18/2
  Add18/1 -> Add19/1
  Gain/1 -> eP/1, Scope/1

== system Reference_CVS/Reference CVSs/Pressures Flows and Volumes/Subsystem5/VolumesForVAD/Subsystem24 ==
  note: y = -0,0069x2 + 1,2813x + 30,375R² = 1
  note: y = -2E-06x 2 + 0,0011x + 0,044
      | R² = 1
  Add18 : Sum
  Add19 : Sum
  Constant20 : Constant  Value=30.375
  Gain : Gain  Gain=1/1000
  Gain2 : Gain  Gain=-0.0069
  Gain3 : Gain  Gain=1.2813
  Product15 : Product
  Scope : Scope
      settings: ActiveDisplayYMinimum=0.07241  ActiveDisplayYMaximum=0.09241  DataLoggingVariableName=ScopeData2
  eLA : Outport
  wires:
  Add18/1 -> Add19/1
  Gain3/1 -> Add18/2
  Product15/1 -> Gain2/1
  Constant20/1 -> Add19/2
  Gain2/1 -> Add18/1
  [HR] -> Product15/1, Product15/2, Gain3/1
  Add19/1 -> Gain/1
  Gain/1 -> eLA/1, Scope/1

== system Reference_CVS/Reference CVSs/Pressures Flows and Volumes/Subsystem5/VolumesForVAD/Subsystem25 ==
  note: y = -0,1479x 2 + 38,021x - 923,75
  Add18 : Sum
  Add19 : Sum
  Constant20 : Constant  Value=-923.75
  Gain : Gain  Gain=1/10000
  Gain2 : Gain  Gain=-0.1479
  Gain3 : Gain  Gain=38.021
  Product15 : Product
  Scope : Scope
      settings: ActiveDisplayYMinimum=0.07241  ActiveDisplayYMaximum=0.09241
  eRA : Outport
  wires:
  Gain/1 -> eRA/1, Scope/1
  Gain2/1 -> Add18/1
  Gain3/1 -> Add18/2
  Product15/1 -> Gain2/1
  Add18/1 -> Add19/1
  Constant20/1 -> Add19/2
  [HR] -> Product15/1, Product15/2, Gain3/1
  Add19/1 -> Gain/1

== system Reference_CVS/Reference CVSs/Pressures Flows and Volumes/Subsystem5/VolumesForVAD/Subsystem26 ==
  note: y = 4,1667x2 + 3041,7x + 12500R² = 1
  note: y = -0,0225x 2 + 8,375x - 211,5
      | R² = 1
  Add18 : Sum
  Add19 : Sum
  Constant20 : Constant  Value=12500
  Gain : Gain  Gain=1/1000
  Gain2 : Gain  Gain=4.1667
  Gain3 : Gain  Gain=3041.7
  Product15 : Product
  Scope : Scope
      settings: ActiveDisplayYMinimum=197.50212  ActiveDisplayYMaximum=216.59303  DataLoggingVariableName=ScopeData2
  gLV : Outport
  wires:
  Add19/1 -> Gain/1
  [HR] -> Gain3/1, Product15/2, Product15/1
  Gain2/1 -> Add18/1
  Constant20/1 -> Add19/2
  Product15/1 -> Gain2/1
  Gain3/1 -> Add18/2
  Add18/1 -> Add19/1
  Gain/1 -> gLV/1, Scope/1

== system Reference_CVS/Reference CVSs/Pressures Flows and Volumes/Subsystem5/VolumesForVAD/Subsystem27 ==
  note: y = 0,25x2 + 1212,5x - 3650R² = 1
  note: y = -0,0092x 2 + 3,2083x - 89,5
      | R² = 1
  Add18 : Sum
  Add19 : Sum
  Constant20 : Constant  Value=-3650
  Gain : Gain  Gain=1/1000
  Gain2 : Gain  Gain=0.25
  Gain3 : Gain  Gain=1212.5
  Product15 : Product
  Scope : Scope
      settings: ActiveDisplayYMinimum=60  ActiveDisplayYMaximum=80  DataLoggingVariableName=ScopeData2
  gVt : Outport
  wires:
  Add19/1 -> Gain/1
  [HR] -> Gain3/1, Product15/2, Product15/1
  Gain2/1 -> Add18/1
  Constant20/1 -> Add19/2
  Product15/1 -> Gain2/1
  Gain3/1 -> Add18/2
  Add18/1 -> Add19/1
  Gain/1 -> gVt/1, Scope/1

== system Reference_CVS/Reference CVSs/Pressures Flows and Volumes/Subsystem5/VolumesForVAD/Subsystem28 ==
  note: y = -0,0208x 2 + 4,7917x - 162,5
  Add18 : Sum
  Add19 : Sum
  Constant20 : Constant  Value=-162.5
  Gain : Gain  Gain=1/10
  Gain2 : Gain  Gain=-0.0208
  Gain3 : Gain  Gain=4.7917
  Product15 : Product
  Scope : Scope
      settings: ActiveDisplayYMinimum=3.9997  ActiveDisplayYMaximum=5.9997  DataLoggingVariableName=ScopeData2
  gP : Outport
  wires:
  Add18/1 -> Add19/1
  Gain3/1 -> Add18/2
  Product15/1 -> Gain2/1
  Constant20/1 -> Add19/2
  Gain2/1 -> Add18/1
  [HR] -> Product15/1, Product15/2, Gain3/1
  Add19/1 -> Gain/1
  Gain/1 -> Scope/1, gP/1

== system Reference_CVS/Reference CVSs/Pressures Flows and Volumes/Subsystem5/VolumesForVAD/eAO resting1 ==
  note: y = 0,5x + 40
  Add19 : Sum
  Constant20 : Constant  Value=40
  Gain1 : Gain  Gain=1/100
  Gain3 : Gain  Gain=0.5
  Scope : Scope
      settings: ActiveDisplayYMinimum=0.50527  ActiveDisplayYMaximum=0.53249  DataLoggingVariableName=ScopeData2
  eAO : Outport
  wires:
  Add19/1 -> Gain1/1
  Gain3/1 -> Add19/1
  Constant20/1 -> Add19/2
  [insan] -> Gain3/1
  Gain1/1 -> eAO/1, Scope/1

== system Reference_CVS/Reference CVSs/Pressures Flows and Volumes/Subsystem5/VolumesForVAD/gao resting1 ==
  note: y = -0,0167x 2 + 3,25x - 45
  Add18 : Sum
  Add19 : Sum
  Constant20 : Constant  Value=-45
  Gain1 : Gain  Gain=1/100
  Gain2 : Gain  Gain=-0.0167
  Gain3 : Gain  Gain=3.25
  Product15 : Product
  Scope : Scope
      settings: ActiveDisplayYMinimum=0.88246  ActiveDisplayYMaximum=1.08246  DataLoggingVariableName=ScopeData2
  gAO : Outport
  wires:
  Gain1/1 -> gAO/1, Scope/1
  Add19/1 -> Gain1/1
  [insan] -> Gain3/1, Product15/2, Product15/1
  Gain2/1 -> Add18/1
  Constant20/1 -> Add19/2
  Product15/1 -> Gain2/1
  Gain3/1 -> Add18/2
  Add18/1 -> Add19/1

== system Reference_CVS/Reference CVSs/Pressures Flows and Volumes/Subsystem5/VolumesForVAD/hf10 ==
  note: y = -0,0069x2 + 1,2813x + 30,375R² = 1
  note: y = -2E-06x 2 + 0,0011x + 0,044
      | R² = 1
  note: y = 0,015x 2 - 2,25x + 301
  Add18 : Sum
  Add19 : Sum
  Constant20 : Constant  Value=301
  Gain : Gain  Gain=1/1000
  Gain2 : Gain  Gain=0.015
  Gain3 : Gain  Gain=-2.25
  Product15 : Product
  Scope : Scope
      settings: ActiveDisplayYMinimum=0.07241  ActiveDisplayYMaximum=0.09241
  eRA : Outport
  wires:
  Add19/1 -> Gain/1
  [HR] -> Gain3/1, Product15/2, Product15/1
  Constant20/1 -> Add19/2
  Add18/1 -> Add19/1
  Product15/1 -> Gain2/1
  Gain3/1 -> Add18/2
  Gain2/1 -> Add18/1
  Gain/1 -> Scope/1, eRA/1

== system Reference_CVS/Reference CVSs/Pressures Flows and Volumes/Subsystem5/VolumesForVAD/hf11 ==
  note: y = -0,0014x 2 + 0,4834x - 14,119
      | R² = 1
  note: y = -0,0073x2 + 26,677x - 591,88R² = 1
  note: y = 0,0079x 2 - 0,7958x + 117,5
  Add18 : Sum
  Add19 : Sum
  Constant20 : Constant  Value=117.5
  Gain1 : Gain  Gain=1/100
  Gain2 : Gain  Gain=0.0079
  Gain3 : Gain  Gain=-0.7958
  Product15 : Product
  Scope : Scope
      settings: ActiveDisplayYMinimum=0.88246  ActiveDisplayYMaximum=1.08246  DataLoggingVariableName=ScopeData2
  gAO : Outport
  wires:
  Gain1/1 -> gAO/1, Scope/1
  Add19/1 -> Gain1/1
  [HR] -> Gain3/1, Product15/2, Product15/1
  Gain2/1 -> Add18/1
  Constant20/1 -> Add19/2
  Product15/1 -> Gain2/1
  Gain3/1 -> Add18/2
  Add18/1 -> Add19/1

== system Reference_CVS/Reference CVSs/Pressures Flows and Volumes/Subsystem5/VolumesForVAD/hf12 ==
  note: y = -0,0008x 2 + 0,2917x + 195,5
      | R² = 1
  note: y = -0,1667x2 + 158,33x + 201100R² = 1
  note: y = 0,0222x 2 - 4,3333x + 230
  Add18 : Sum
  Add19 : Sum
  Constant20 : Constant  Value=230
  Gain2 : Gain  Gain=0.0222
  Gain3 : Gain  Gain=-4.3333
  Product15 : Product
  Scope : Scope
      settings: ActiveDisplayYMinimum=109.99968  ActiveDisplayYMaximum=309.99968  DataLoggingVariableName=ScopeData2
  gRV : Outport
  wires:
  Add19/1 -> Scope/1, gRV/1
  Add18/1 -> Add19/1
  Gain3/1 -> Add18/2
  Product15/1 -> Gain2/1
  Constant20/1 -> Add19/2
  Gain2/1 -> Add18/1
  [HR] -> Product15/1, Product15/2, Gain3/1

== system Reference_CVS/Reference CVSs/Pressures Flows and Volumes/Subsystem5/VolumesForVAD/hf7 ==
  note: y = 0,0054x 2 - 1,6458x + 199,25
      | R² = 1
  note: y = 0,0167x 2 - 3,1667x + 240
  Add18 : Sum
  Add19 : Sum
  Constant20 : Constant  Value=240
  Gain : Gain  Gain=1/1000
  Gain2 : Gain  Gain=0.0167
  Gain3 : Gain  Gain=-3.1667
  Product15 : Product
  Scope : Scope
      settings: ActiveDisplayYMinimum=0.01994  ActiveDisplayYMaximum=0.21994  DataLoggingVariableName=ScopeData2
  eP : Outport
  wires:
  Add19/1 -> Gain/1
  [HR] -> Gain3/1, Product15/2, Product15/1
  Gain2/1 -> Add18/1
  Constant20/1 -> Add19/2
  Product15/1 -> Gain2/1
  Gain3/1 -> Add18/2
  Add18/1 -> Add19/1
  Gain/1 -> eP/1, Scope/1

== system Reference_CVS/Reference CVSs/Pressures Flows and Volumes/Subsystem5/VolumesForVAD/hf8 ==
  note: y = -1E-16x 2 + 0,6667x - 3E-13
  Add18 : Sum
  Add19 : Sum
  Constant20 : Constant  Value=-3e-13
  Display : Display
  Gain1 : Gain  Gain=1/10000
  Gain2 : Gain  Gain=-1e-16
  Gain3 : Gain  Gain=0.6667
  Product15 : Product
  Scope : Scope
      settings: ActiveDisplayYMinimum=0.00132  ActiveDisplayYMaximum=0.00154  DataLoggingVariableName=ScopeData2
  eV : Outport
  wires:
  Gain1/1 -> eV/1, Display/1, Scope/1
  Add19/1 -> Gain1/1
  [HR] -> Gain3/1, Product15/2, Product15/1
  Gain2/1 -> Add18/1
  Constant20/1 -> Add19/2
  Product15/1 -> Gain2/1
  Gain3/1 -> Add18/2
  Add18/1 -> Add19/1

== system Reference_CVS/Reference CVSs/Pressures Flows and Volumes/Subsystem5/VolumesForVAD/hf9 ==
  note: y = 0,0167x 2 - 2,8333x + 220
  note: y = -2E-06x 2 + 0,0011x + 0,044
      | R² = 1
  Add18 : Sum
  Add19 : Sum
  Constant20 : Constant  Value=220
  Gain : Gain  Gain=1/1000
  Gain2 : Gain  Gain=0.0167
  Gain3 : Gain  Gain=-2.8333
  Product15 : Product
  Scope : Scope
      settings: ActiveDisplayYMinimum=0.07241  ActiveDisplayYMaximum=0.09241  DataLoggingVariableName=ScopeData2
  eLA : Outport
  wires:
  Gain/1 -> Scope/1, eLA/1
  Add19/1 -> Gain/1
  [HR] -> Gain3/1, Product15/2, Product15/1
  Gain2/1 -> Add18/1
  Constant20/1 -> Add19/2
  Product15/1 -> Gain2/1
  Gain3/1 -> Add18/2
  Add18/1 -> Add19/1

== system Reference_CVS/Reference CVSs/Pressures Flows and Volumes/Subsystem5/VolumesForVAD/hfao1 ==
  note: y = 0,0271x2 - 8,2292x + 5621,2R² = 1
  note: y = 0,0003x2 - 0,0823x + 56,212R² = 1
  note: y = 3E-06x2 - 0,0008x + 0,5621R² = 1
  Add18 : Sum
  Add19 : Sum
  Constant20 : Constant  Value=0.5621
  Gain2 : Gain  Gain=0.000003
  Gain3 : Gain  Gain=-0.0008
  Product15 : Product
  Scope : Scope
      settings: ActiveDisplayYMinimum=0.50527  ActiveDisplayYMaximum=0.53249  DataLoggingVariableName=ScopeData2
  eAO : Outport
  wires:
  Add19/1 -> eAO/1, Scope/1
  Add18/1 -> Add19/1
  Gain3/1 -> Add18/2
  Product15/1 -> Gain2/1
  Constant20/1 -> Add19/2
  Gain2/1 -> Add18/1
  [HR] -> Product15/1, Product15/2, Gain3/1

== system Reference_CVS/Reference CVSs/eRV/RV_e_min/c_RV/PID ==
  s : Inport
  LTI System : cstblocks/LTI System  sys=tfa  IC=[]
  PID Controller : simulink/Continuous/PID Controller  Controller=PID  Form=Parallel  TimeDomain=Continuous-time  SampleTime=-1  IntegratorMethod=Forward Euler  FilterMethod=Forward Euler  ControllerParametersSource=internal  P=0  I=0.336541519886425  D=0  UseFilter=on  N=100  TunerSelectOption=Transfer Function Based (PID Tuner App)  InitialConditionSource=internal  InitialConditionForIntegrator=0  InitialConditionForFilter=0  DifferentiatorICPrevScaledInput=0  ExternalReset=none  TrackingMode=off  Kt=1  LimitOutput=off  UpperSaturationLimit=inf  LowerSaturationLimit=-inf  LinearizeAsGain=on  AntiWindupMode=none  Kb=1  POutMin=[]  POutMax=[]  IOutMin=[]  IOutMax=[]  DOutMin=[]  DOutMax=[]  NOutMin=[]  NOutMax=[]  SumOutMin=[]  SumOutMax=[]  SaturationOutMin=[]  SaturationOutMax=[]  PParamMin=[]  PParamMax=[]  IParamMin=[]  IParamMax=[]  DParamMin=[]  DParamMax=[]  NParamMin=[]  NParamMax=[]  KbParamMin=[]  KbParamMax=[]  KtParamMin=[]  KtParamMax=[]  KbOutMin=[]  KbOutMax=[]  KtOutMin=[]  KtOutMax=[]  IntegratorOutMin=[]  IntegratorOutMax=[]  FilterOutMin=[]  FilterOutMax=[]  SumI1OutMin=[]  SumI1OutMax=[]  SumI2OutMin=[]  SumI2OutMax=[]  SumI3OutMin=[]  SumI3OutMax=[]  SumI4OutMin=[]  SumI4OutMax=[]  SumDOutMin=[]  SumDOutMax=[]  DifferentiatorOutMin=[]  DifferentiatorOutMax=[]  FilterDiffOutCoefMin=[]  FilterDiffOutCoefMax=[]  ReciprocalOutMin=[]  ReciprocalOutMax=[]  SumDenOutMin=[]  SumDenOutMax=[]  SumNumOutMin=[]  SumNumOutMax=[]  DivideOutMin=[]  DivideOutMax=[]  IntegratorContinuousStateAttributes=''  IntegratorStateMustResolveToSignalObject=off  IntegratorRTWStateStorageClass=Auto  FilterContinuousStateAttributes=''  FilterStateMustResolveToSignalObject=off  FilterRTWStateStorageClass=Auto  ParallelPVariant=InternalParameters  IdealPVariant=Disabled  IVariant=InternalParameters  DVariant=InternalParameters  IntegratorVariant=Continuous  SatVariant=Disabled  AWVariant=Passthrough  PCopyVariant=Disabled  TRVariant=Disabled  FdbkBlocksVariant=Forward  IdealPFdbkVariant=Disabled  SatFdbkVariant=Disabled  DerivativeFilterVariant=ContFilter  NVariant=InternalParameters  NCopyVariant=Disabled  FilterICVariant=InternalICsFilter  IntegratorICVariant=InternalICs  ExternalResetVariant=Disabled  TRSumVariant=Passthrough  SumFdbkVariant=Disabled  SumVariant=Sum_PID
  Sum1 : Sum  Inputs=|+-
  To Workspace : ToWorkspace  VariableName=input  SampleTime=-1
  To Workspace1 : ToWorkspace  VariableName=output  SampleTime=-1
  E : Outport  VectorParamsAs1DForOutWhenUnconnected=off
  wires:
  PID Controller/1 -> To Workspace/1, LTI System/1
  s/1 -> Sum1/1
  Sum1/1 -> PID Controller/1
  LTI System/1 -> Sum1/2, E/1, To Workspace1/1

== system Reference_CVS/Reference CVSs/eRV/RV_e_min/real_c_RV/PID ==
  s : Inport
  LTI System : cstblocks/LTI System  sys=tfa  IC=[]
  PID Controller : simulink/Continuous/PID Controller  Controller=PID  Form=Parallel  TimeDomain=Continuous-time  SampleTime=-1  IntegratorMethod=Forward Euler  FilterMethod=Forward Euler  ControllerParametersSource=internal  P=0  I=0.336541519886425  D=0  UseFilter=on  N=100  TunerSelectOption=Transfer Function Based (PID Tuner App)  InitialConditionSource=internal  InitialConditionForIntegrator=0  InitialConditionForFilter=0  DifferentiatorICPrevScaledInput=0  ExternalReset=none  TrackingMode=off  Kt=1  LimitOutput=off  UpperSaturationLimit=inf  LowerSaturationLimit=-inf  LinearizeAsGain=on  AntiWindupMode=none  Kb=1  POutMin=[]  POutMax=[]  IOutMin=[]  IOutMax=[]  DOutMin=[]  DOutMax=[]  NOutMin=[]  NOutMax=[]  SumOutMin=[]  SumOutMax=[]  SaturationOutMin=[]  SaturationOutMax=[]  PParamMin=[]  PParamMax=[]  IParamMin=[]  IParamMax=[]  DParamMin=[]  DParamMax=[]  NParamMin=[]  NParamMax=[]  KbParamMin=[]  KbParamMax=[]  KtParamMin=[]  KtParamMax=[]  KbOutMin=[]  KbOutMax=[]  KtOutMin=[]  KtOutMax=[]  IntegratorOutMin=[]  IntegratorOutMax=[]  FilterOutMin=[]  FilterOutMax=[]  SumI1OutMin=[]  SumI1OutMax=[]  SumI2OutMin=[]  SumI2OutMax=[]  SumI3OutMin=[]  SumI3OutMax=[]  SumI4OutMin=[]  SumI4OutMax=[]  SumDOutMin=[]  SumDOutMax=[]  DifferentiatorOutMin=[]  DifferentiatorOutMax=[]  FilterDiffOutCoefMin=[]  FilterDiffOutCoefMax=[]  ReciprocalOutMin=[]  ReciprocalOutMax=[]  SumDenOutMin=[]  SumDenOutMax=[]  SumNumOutMin=[]  SumNumOutMax=[]  DivideOutMin=[]  DivideOutMax=[]  IntegratorContinuousStateAttributes=''  IntegratorStateMustResolveToSignalObject=off  IntegratorRTWStateStorageClass=Auto  FilterContinuousStateAttributes=''  FilterStateMustResolveToSignalObject=off  FilterRTWStateStorageClass=Auto  ParallelPVariant=InternalParameters  IdealPVariant=Disabled  IVariant=InternalParameters  DVariant=InternalParameters  IntegratorVariant=Continuous  SatVariant=Disabled  AWVariant=Passthrough  PCopyVariant=Disabled  TRVariant=Disabled  FdbkBlocksVariant=Forward  IdealPFdbkVariant=Disabled  SatFdbkVariant=Disabled  DerivativeFilterVariant=ContFilter  NVariant=InternalParameters  NCopyVariant=Disabled  FilterICVariant=InternalICsFilter  IntegratorICVariant=InternalICs  ExternalResetVariant=Disabled  TRSumVariant=Passthrough  SumFdbkVariant=Disabled  SumVariant=Sum_PID
  Sum1 : Sum  Inputs=|+-
  To Workspace : ToWorkspace  VariableName=input  SampleTime=-1
  To Workspace1 : ToWorkspace  VariableName=output  SampleTime=-1
  E : Outport  VectorParamsAs1DForOutWhenUnconnected=off
  wires:
  LTI System/1 -> To Workspace1/1, E/1, Sum1/2
  Sum1/1 -> PID Controller/1
  s/1 -> Sum1/1
  PID Controller/1 -> LTI System/1, To Workspace/1

== matlab function Reference_CVS/Reference CVSs/Pressures Flows and Volumes/Subsystem5/VolumesForVAD/MATLAB Function ==
  data: u input; y output; HR input
function y = fcn(u,HR)

tbeatlol =60/HR;
y = mod(u,tbeatlol);
end

== matlab function Reference_CVS/Reference CVSs/Pressures Flows and Volumes/MATLAB Function ==
  data: u input; y output; HR input
function y = fcn(u,HR)

tbeatlol =60/HR;
y = mod(u,tbeatlol);
end
